simulink model "ProdSystem_QrAssumptionsAndCosts"  (R2015a)
settings: Solver=ode45  SolverMode=SingleTasking  StartTime=0  StopTime=100000000  RelTol=1e-3
libraries: simeventslib x12, simulink x1
settings Model: CovSFcnEnable=off  Creator=AnotherUser  LastModifiedBy=gthiers3
settings OptimizationCC: BlockReduction=off  BooleanDataType=off
settings DebuggingCC: SaveWithParameterizedLinksMsg=none  UnderspecifiedInitializationDetection=Classic  MergeDetectMultiDrivingBlocksExec=none  SignalResolutionControl=TryResolveAllWithWarning
settings HardwareCC: TargetUnknown=on

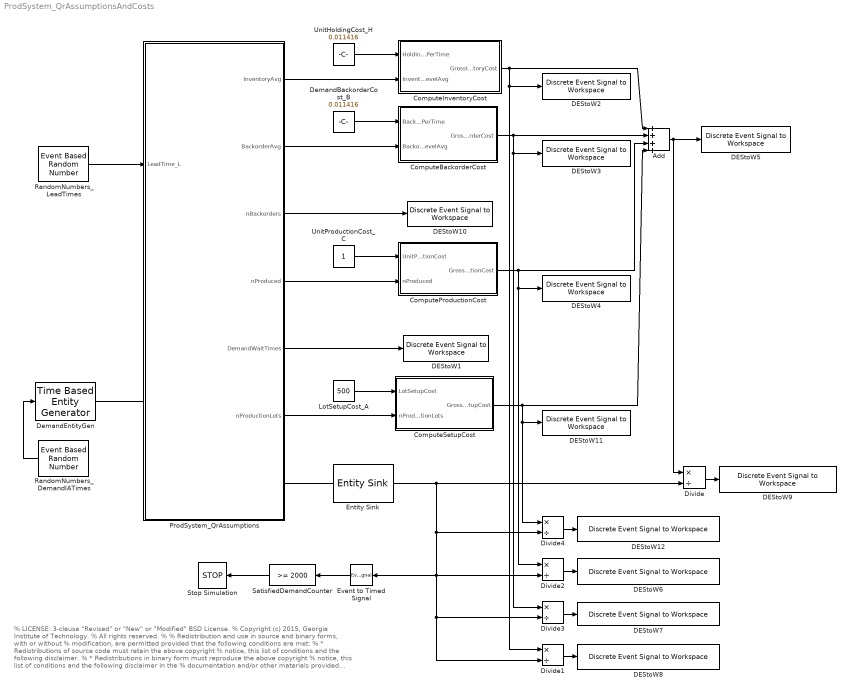
== system ProdSystem_QrAssumptionsAndCosts ==
  note: % LICENSE: 3-clause "Revised" or "New" or "Modified" BSD License.
      | % Copyright (c) 2015, Georgia Institute of Technology.
      | % All rights reserved.
      | %
      | % Redistribution and use in source and binary forms, with or without
      | % modification, are permitted provided that the following conditions are met:
      | % * Redistributions of source code must retain the above copyright
      | % notice, this list of conditions and the following disclaimer.
      | % * Redistributions in binary form must reproduce the above copyright
      | % notice, this list of conditions and the following disclaimer in the
      | % documentation and/or other materials provided with the distribution.
      | % * Neither the name of the Georgia Institute of Technology nor the
      | % names of its contributors may be used to endorse or promote products
      | % derived from this software without specific prior written permission.
      | %
      | % THIS SOFTWARE IS PROVIDED BY THE COPYRIGHT HOLDERS AND CONTRIBUTORS "AS IS" AND
      | % ANY EXPRESS OR IMPLIED WARRANTIES, INCLUDING, BUT NOT LIMITED TO, THE IMPLIED
      | % WARRANTIES OF MERCHANTABILITY AND FITNESS FOR A PARTICULAR PURPOSE ARE
      | % DISCLAIMED. IN NO EVENT SHALL THE GEORGIA INSTITUTE OF TECHNOLOGY BE LIABLE FOR
      | % ANY DIRECT, INDIRECT, INCIDENTAL, SPECIAL, EXEMPLARY, OR CONSEQUENTIAL DAMAGES
      | % (INCLUDING, BUT NOT LIMITED TO, PROCUREMENT OF SUBSTITUTE GOODS OR SERVICES;
      | % LOSS OF USE, DATA, OR PROFITS; OR BUSINESS INTERRUPTION) HOWEVER CAUSED AND
      | % ON ANY THEORY OF LIABILITY, WHETHER IN CONTRACT, STRICT LIABILITY, OR TORT
      | % (INCLUDING NEGLIGENCE OR OTHERWISE) ARISING IN ANY WAY OUT OF THE USE OF THIS
      | % SOFTWARE, EVEN IF ADVISED OF THE POSSIBILITY OF SUCH DAMAGE.
  Add : Sum  Inputs=++++
  ComputeBackorderCost : Subsystem
  ComputeInventoryCost : Subsystem
  ComputeProductionCost : Subsystem
  ComputeSetupCost : Subsystem
  DEStoW1 : simeventslib/SimEvents Sinks/Discrete Event Signal to Workspace  VariableName=DemandWaitTimes  SaveFormat=Structure With Time  isMonitorOnly=off  isRecordIC=off
  DEStoW10 : simeventslib/SimEvents Sinks/Discrete Event Signal to Workspace  VariableName=nBackorders  SaveFormat=Structure With Time  isMonitorOnly=off  isRecordIC=off
  DEStoW11 : simeventslib/SimEvents Sinks/Discrete Event Signal to Workspace  VariableName=GrossSetupCost  SaveFormat=Structure With Time  isMonitorOnly=off  isRecordIC=off
  DEStoW12 : simeventslib/SimEvents Sinks/Discrete Event Signal to Workspace  VariableName=GrossSetupCost_PerSatDmd  SaveFormat=Structure With Time  isMonitorOnly=off  isRecordIC=off
  DEStoW2 : simeventslib/SimEvents Sinks/Discrete Event Signal to Workspace  VariableName=GrossInventoryCost  SaveFormat=Structure With Time  isMonitorOnly=off  isRecordIC=off
  DEStoW3 : simeventslib/SimEvents Sinks/Discrete Event Signal to Workspace  VariableName=GrossBackorderCost  SaveFormat=Structure With Time  isMonitorOnly=off  isRecordIC=off
  DEStoW4 : simeventslib/SimEvents Sinks/Discrete Event Signal to Workspace  VariableName=GrossProductionCost  SaveFormat=Structure With Time  isMonitorOnly=off  isRecordIC=off
  DEStoW5 : simeventslib/SimEvents Sinks/Discrete Event Signal to Workspace  VariableName=GrossCost  SaveFormat=Structure With Time  isMonitorOnly=off  isRecordIC=off
  DEStoW6 : simeventslib/SimEvents Sinks/Discrete Event Signal to Workspace  VariableName=GrossProductionCost_PerSatDmd  SaveFormat=Structure With Time  isMonitorOnly=off  isRecordIC=off
  DEStoW7 : simeventslib/SimEvents Sinks/Discrete Event Signal to Workspace  VariableName=GrossBackorderCost_PerSatDmd  SaveFormat=Structure With Time  isMonitorOnly=off  isRecordIC=off
  DEStoW8 : simeventslib/SimEvents Sinks/Discrete Event Signal to Workspace  VariableName=GrossInventoryCost_PerSatDmd  SaveFormat=Structure With Time  isMonitorOnly=off  isRecordIC=off
  DEStoW9 : simeventslib/SimEvents Sinks/Discrete Event Signal to Workspace  VariableName=GrossCost_PerSatDmd  SaveFormat=Structure With Time  isMonitorOnly=off  isRecordIC=off
  DemandBackorderCost_B : Constant  Value=0.011416
  DemandEntityGen : TimeBasedEntityGenerator  GenerateEntitiesUpon=Intergeneration time from port t  GenerateEntityAtSimulationStart=off
  Divide{,1..4} (5 alike) : Product  Inputs=*/
  Entity Sink : EntitySink  StatNumberArrived=on
  Event to Timed Signal : EventToTimedSignal
  LotSetupCost_A : Constant  Value=500
  ProdSystem_QrAssumptions : Subsystem  mask{LotSizeQ=37, ReorderPointR=12}
      mask prompts: LotSizeQ "Lot Size Q:"; ReorderPointR "Reorder Point R:"
      mask TypeOptions LotSizeQ: LotSize_Q/Value
      mask Callback LotSizeQ:
      | %% LotSizeQ is defined as a mask parameter
      | qStr = get_param(gcbh, 'LotSizeQ');
      | qInt = int32(str2double(qStr));  %Enforce integer
      | if qInt < 1  %str2double returns NaN for non-numerical input, and int32 returns 0 for NaN
      |     error('Invalid input for LotSizeQ');
      | end
      | set_param(gcbh, 'LotSizeQ', num2str(qInt));  %Correct any non-integer value
      | 
      | 
      | %% ReorderPointR is defined as a mask parameter
      | rStr = get_param(gcbh, 'ReorderPointR');
      | rInt = int32(str2double(rStr));  %Enforce integer
      | if rInt < 1  %str2double returns NaN for non-numerical input, and int32 returns 0 for NaN
      |     error('Invalid input for ReorderPointR');
      | end
      | set_param(gcbh, 'ReorderPointR', num2str(rInt));  %Correct any non-integer value
      | 
      | 
      | %% Get path of TimeBasedFunctionCallGenerator
      | prodSysPath = [gcs '/' get(gcbh,'Name')];
      | timeBasedFcnCallGenPath = [prodSysPath '/FcnCallGen_T0'];
      | %% Set number of fcn calls at T0
      | if qInt <= rInt
      |     set_param(timeBasedFcnCallGenPath, 'NumberOfEventsPerPeriod', num2str(rInt+1));
      | else
      |     set_param(timeBasedFcnCallGenPath, 'NumberOfEventsPerPeriod', num2str(1));
      | end
      mask TypeOptions ReorderPointR: ReorderPoint_R/Value
      mask Callback ReorderPointR:
      | %% LotSizeQ is defined as a mask parameter
      | qStr = get_param(gcbh, 'LotSizeQ');
      | qInt = int32(str2double(qStr));  %Enforce integer
      | if qInt < 1  %str2double returns NaN for non-numerical input, and int32 returns 0 for NaN
      |     error('Invalid input for LotSizeQ');
      | end
      | set_param(gcbh, 'LotSizeQ', num2str(qInt));  %Correct any non-integer value
      | 
      | 
      | %% ReorderPointR is defined as a mask parameter
      | rStr = get_param(gcbh, 'ReorderPointR');
      | rInt = int32(str2double(rStr));  %Enforce integer
      | if rInt < 1  %str2double returns NaN for non-numerical input, and int32 returns 0 for NaN
      |     error('Invalid input for ReorderPointR');
      | end
      | set_param(gcbh, 'ReorderPointR', num2str(rInt));  %Correct any non-integer value
      | 
      | 
      | %% Get path of TimeBasedFunctionCallGenerator
      | prodSysPath = [gcs '/' get(gcbh,'Name')];
      | timeBasedFcnCallGenPath = [prodSysPath '/FcnCallGen_T0'];
      | %% Set number of fcn calls at T0
      | if qInt <= rInt
      |     set_param(timeBasedFcnCallGenPath, 'NumberOfEventsPerPeriod', num2str(rInt+1));
      | else
      |     set_param(timeBasedFcnCallGenPath, 'NumberOfEventsPerPeriod', num2str(1));
      | end
      mask DialogControl DescTextVar Prompt: (1) Demands occur randomly and one at a time, (2) Demand which is not filled immediately is backordered, (3) Replenishment lead times are known and deterministic (relaxed here - they can be random, or deterministic by choosing the normal distribution with stdev=eps, which is as close to zero as possible), (4) When the inventory position (not the inventory on-hand) drops to the reorder point R, immediately reorder a lot of size Q, (5) One version of the Qr model constrains the number of replenishment orders per time period, *but such a constraint is not implemented here*.
  RandomNumbers_DemandIATimes : EventBasedRandomNumber  Distribution=Gamma  meanExp=8.76  scaleGam=62.5714  meanNorm=0.73  stdNorm=0.32647  scaleLogn=3.6885  shapeLogn=0.42699  Seed=63378
  RandomNumbers_LeadTimes : EventBasedRandomNumber  Distribution=Gamma  meanExp=8.76  scaleGam=1.5561e-11  shapeGam=70368744177664  meanNorm=600  stdNorm=eps  scaleLogn=11.0128  shapeLogn=1.2905e-07  Seed=7493
  SatisfiedDemandCounter : simulink/Logic and Bit Operations/Compare To Constant  relop=>=  const=2000  OutDataTypeStr=boolean
  Stop Simulation : Stop
  UnitHoldingCost_H : Constant  Value=0.011416
  UnitProductionCost_C : Constant
  wires:
  RandomNumbers_DemandIATimes/1 -> DemandEntityGen/1
  Add/1 -> DEStoW5/1, Divide/1
  ProdSystem_QrAssumptions/5(DemandWaitTimes) -> DEStoW1/1
  Divide/1 -> DEStoW9/1
  Divide1/1 -> DEStoW8/1
  Divide2/1 -> DEStoW6/1
  Divide3/1 -> DEStoW7/1
  Entity Sink/1 -> Divide4/2, Divide2/2, Event to Timed Signal/1, Divide1/2, Divide3/2, Divide/2
  RandomNumbers_LeadTimes/1 -> ProdSystem_QrAssumptions/1(LeadTime_L)
  ComputeInventoryCost/1(GrossInventoryCost) -> Divide1/1, DEStoW2/1, Add/1
  UnitHoldingCost_H/1 -> ComputeInventoryCost/1(HoldingCost_PerUnitPerTime)
  ProdSystem_QrAssumptions/1(InventoryAvg) -> ComputeInventoryCost/2(InventoryLevelAvg)
  ComputeBackorderCost/1(GrossBackorderCost) -> Divide3/1, DEStoW3/1, Add/2
  ProdSystem_QrAssumptions/2(BackorderAvg) -> ComputeBackorderCost/2(BackorderLevelAvg)
  DemandBackorderCost_B/1 -> ComputeBackorderCost/1(BackorderCost_PerUnitPerTime)
  ComputeProductionCost/1(GrossProductionCost) -> Divide2/1, DEStoW4/1, Add/3
  ProdSystem_QrAssumptions/4(nProduced) -> ComputeProductionCost/2(nProduced)
  UnitProductionCost_C/1 -> ComputeProductionCost/1(UnitProductionCost)
  ProdSystem_QrAssumptions/3(nBackorders) -> DEStoW10/1
  ProdSystem_QrAssumptions/6(nProductionLots) -> ComputeSetupCost/2(nProductionLots)
  LotSetupCost_A/1 -> ComputeSetupCost/1(LotSetupCost)
  ComputeSetupCost/1(GrossSetupCost) -> Divide4/1, DEStoW11/1, Add/4
  Divide4/1 -> DEStoW12/1
  Event to Timed Signal/1 -> SatisfiedDemandCounter/1
  SatisfiedDemandCounter/1 -> Stop Simulation/1
  connections:
  DemandEntityGen/RConn1 -- ProdSystem_QrAssumptions/LConn1
  ProdSystem_QrAssumptions/RConn1 -- Entity Sink/LConn1

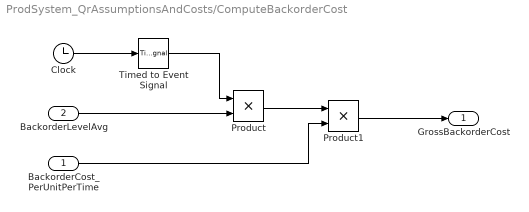
== system ProdSystem_QrAssumptionsAndCosts/ComputeBackorderCost ==
  BackorderCost_PerUnitPerTime : Inport
  BackorderLevelAvg : Inport  Port=2
  Clock : Clock
  Product : Product
  Product1 : Product
  Timed to Event Signal : TimedToEventSignal
  GrossBackorderCost : Outport
  wires:
  BackorderLevelAvg/1 -> Product/2
  Product/1 -> Product1/1
  BackorderCost_PerUnitPerTime/1 -> Product1/2
  Product1/1 -> GrossBackorderCost/1
  Clock/1 -> Timed to Event Signal/1
  Timed to Event Signal/1 -> Product/1

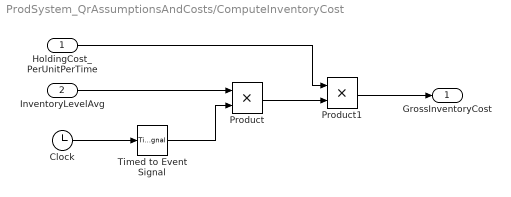
== system ProdSystem_QrAssumptionsAndCosts/ComputeInventoryCost ==
  HoldingCost_PerUnitPerTime : Inport
  InventoryLevelAvg : Inport  Port=2
  Clock : Clock
  Product : Product
  Product1 : Product
  Timed to Event Signal : TimedToEventSignal
  GrossInventoryCost : Outport
  wires:
  Clock/1 -> Timed to Event Signal/1
  Timed to Event Signal/1 -> Product/2
  InventoryLevelAvg/1 -> Product/1
  Product/1 -> Product1/2
  HoldingCost_PerUnitPerTime/1 -> Product1/1
  Product1/1 -> GrossInventoryCost/1

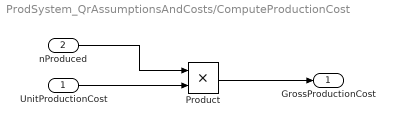
== system ProdSystem_QrAssumptionsAndCosts/ComputeProductionCost ==
  UnitProductionCost : Inport
  nProduced : Inport  Port=2
  Product : Product
  GrossProductionCost : Outport
  wires:
  nProduced/1 -> Product/1
  UnitProductionCost/1 -> Product/2
  Product/1 -> GrossProductionCost/1

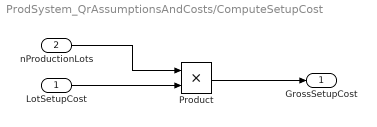
== system ProdSystem_QrAssumptionsAndCosts/ComputeSetupCost ==
  LotSetupCost : Inport
  nProductionLots : Inport  Port=2
  Product : Product
  GrossSetupCost : Outport
  wires:
  nProductionLots/1 -> Product/1
  LotSetupCost/1 -> Product/2
  Product/1 -> GrossSetupCost/1

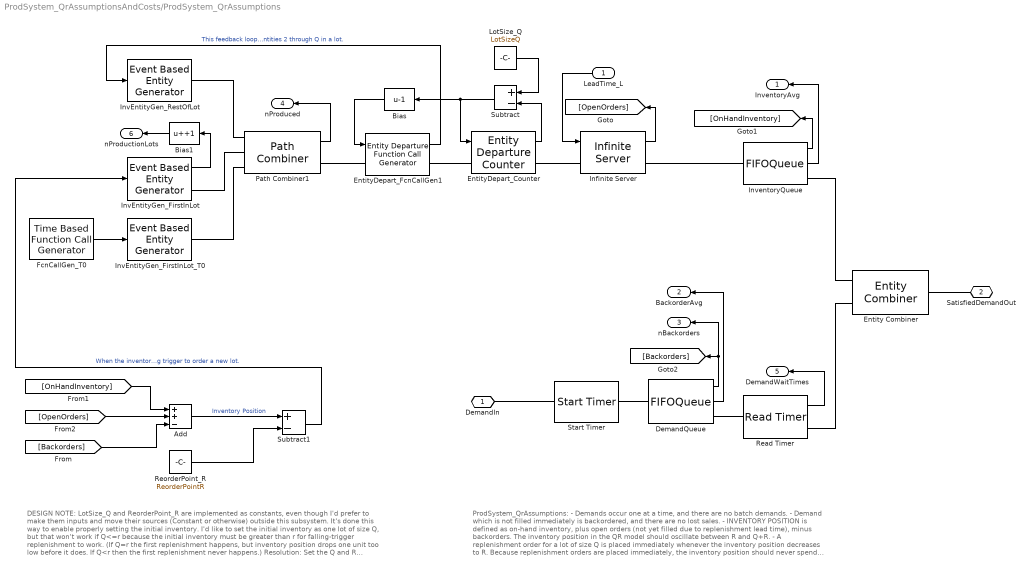
== system ProdSystem_QrAssumptionsAndCosts/ProdSystem_QrAssumptions ==
  note: DESIGN NOTE:  LotSize_Q and ReorderPoint_R are implemented as constants, even
      | though I'd prefer to make them inputs and move their sources (Constant or otherwise)
      | outside this subsystem.  It's done this way to enable properly setting the initial inventory.
      | I'd like to set the initial inventory as one lot of size Q, but that won't work if Q<=r because
      | the initial inventory must be greater than r for falling-trigger replenishment to work.  (If Q=r
      | the first replenishment happens, but inventory position drops one unit too low before it
      | does.  If Q<r then the first replenishment never happens.)
      |
      | Resolution:  Set the Q and R constant blocks through a mask, and use a mask callback
      | function to ensure that the initial inventory level is strictly greater than the reorder point.
  note: ProdSystem_QrAssumptions:
      |
      | - Demands occur one at a time, and there are no batch demands.
      |
      | - Demand which is not filled immediately is backordered, and there are no lost sales.
      |
      | - INVENTORY POSITION is defined as on-hand inventory, plus open orders (not yet filled due to
      | replenishment lead time), minus backorders. The inventory position in the QR model should
      | oscillate between R and Q+R.
      |
      | - A replenishment order for a lot of size Q is placed immediately whenever the inventory position
      | decreases to R. Because replenishment orders are placed immediately, the inventory position
      | should never spend time at level R, but rather jump immediately to Q+R upon decreasing to R.
      |
      | - Production and delivery of replenishment orders are NOT instantaneous, but rather require a
      | fixed and known replenishment lead time. The "fixed and known" assumption is relaxed in the
      | simulation model - replenishment lead times can be random, or made deterministic by choosing
      | the normal distribution with stdev=eps, which is as close to zero as possible.
  LeadTime_L : Inport
  Add : Sum  Inputs=++-
  Bias : Bias  Bias=-1
  Bias1 : Bias  Bias=+1
  DemandQueue : FIFOQueue  Capacity=Inf  StatNumberInBlock=on  StatAverageQueueLength=on
      settings: OutputPortMap=o1,o3
  Entity Combiner : EntityCombiner  NumberInputPorts=2  AttributeAccessibility=off  TimerAccessibility=off
  EntityDepart_Counter : EntityDepartureCounter  NumberDepartedToSignal=on  NumberDepartedToAttribute=off  CounterResetTypeOption=Trigger from port tr  CounterResetEdgeOption=Falling
  EntityDepart_FcnCallGen1 : EntityDepartureFunctionCallGenerator  EnableE1Port=on
  FcnCallGen_T0 : TimeBasedFunctionCallGenerator  EventGenerationMode=Only at simulation start
  Infinite Server : InfiniteServer  ServiceTimeFrom=Signal port t  StatNumberInBlock=on
      settings: OutputPortMap=o1
  InvEntityGen_FirstInLot : EventBasedEntityGenerator  GenerateEntitiesUpon=Trigger from port tr  SignalEdgeType=Falling  StatNumberDeparted=on
  InvEntityGen_FirstInLot_T0 : EventBasedEntityGenerator  GenerateEntitiesUpon=Function call from port fcn
  InvEntityGen_RestOfLot : EventBasedEntityGenerator  GenerateEntitiesUpon=Function call from port fcn
  InventoryQueue : FIFOQueue  Capacity=Inf  StatNumberInBlock=on  StatAverageQueueLength=on
      settings: OutputPortMap=o1,o3
  LotSize_Q : Constant  Value=LotSizeQ
  Path Combiner1 : PathCombiner  StatNumberDeparted=on
  Read Timer : ReadTimer  StatTimeElapsed=on
      settings: OutputPortMap=o2
  ReorderPoint_R : Constant  Value=ReorderPointR
  Start Timer : StartTimer
  Subtract : Sum  Inputs=+-
  Subtract1 : Sum  Inputs=+-
  DemandIn : PMIOPort  Port=1  Side=Left
  SatisfiedDemandOut : PMIOPort  Port=2  Side=Right
  InventoryAvg : Outport
  BackorderAvg : Outport  Port=2
  nBackorders : Outport  Port=3
  nProduced : Outport  Port=4
  DemandWaitTimes : Outport  Port=5
  nProductionLots : Outport  Port=6
  wires:
  LeadTime_L/1 -> Infinite Server/1
  DemandQueue/2 -> BackorderAvg/1
  Read Timer/1 -> DemandWaitTimes/1
  InventoryQueue/2 -> InventoryAvg/1
  Infinite Server/1 -> [OpenOrders]
  InventoryQueue/1 -> [OnHandInventory]
  DemandQueue/1 -> nBackorders/1, [Backorders]
  [OpenOrders] -> Add/2
  [OnHandInventory] -> Add/1
  [Backorders] -> Add/3
  EntityDepart_FcnCallGen1/1 -> InvEntityGen_RestOfLot/1  "This feedback loop produces entities 2 through Q in a lot."
  Subtract/1 -> EntityDepart_Counter/1, Bias/1
  FcnCallGen_T0/1 -> InvEntityGen_FirstInLot_T0/1
  Bias/1 -> EntityDepart_FcnCallGen1/1
  EntityDepart_Counter/1 -> Subtract/2
  LotSize_Q/1 -> Subtract/1
  Path Combiner1/1 -> nProduced/1
  Bias1/1 -> nProductionLots/1
  InvEntityGen_FirstInLot/1 -> Bias1/1
  Add/1 -> Subtract1/1  "Inventory Position"
  Subtract1/1 -> InvEntityGen_FirstInLot/1  "When the inventory position decreases to the reorder point,  that serves as a falling trigger to order a new lot."
  ReorderPoint_R/1 -> Subtract1/2
  connections:
  Read Timer/RConn1 -- Entity Combiner/LConn2
  Entity Combiner/RConn1 -- SatisfiedDemandOut/RConn1
  DemandQueue/LConn1 -- Start Timer/RConn1
  DemandQueue/RConn1 -- Read Timer/LConn1
  InventoryQueue/RConn1 -- Entity Combiner/LConn1
  Path Combiner1/LConn1 -- InvEntityGen_RestOfLot/RConn1
  Path Combiner1/LConn3 -- InvEntityGen_FirstInLot_T0/RConn1
  Path Combiner1/LConn2 -- InvEntityGen_FirstInLot/RConn1
  Path Combiner1/RConn1 -- EntityDepart_FcnCallGen1/LConn1
  EntityDepart_FcnCallGen1/RConn1 -- EntityDepart_Counter/LConn1
  DemandIn/RConn1 -- Start Timer/LConn1
  EntityDepart_Counter/RConn1 -- Infinite Server/LConn1
  Infinite Server/RConn1 -- InventoryQueue/LConn1
